simulink model "seat_heating_control"  (R2023b)
settings: Solver=FixedStepDiscrete  StartTime=0.0  StopTime=10.0  FixedStep=0.01  RelTol=1e-3
values from neighbouring files (symbols this model uses):
  RTE_OK = 0    [init.m]
  TemperatureStage1 = Simulink.Parameter    [init.m]
  TemperatureStage2 = Simulink.Parameter    [init.m]
  TemperatureStage3 = Simulink.Parameter    [init.m]
undefined symbols (not defined in the file or in its folder): EnumPowerState
settings Model: Creator=nabilekhoury  LastModifiedBy=developer
settings SolverCC: AlgebraicLoopSolver=TrustRegion
settings DataIOCC: SaveFormat=StructureWithTime
settings OptimizationCC: DefaultParameterBehavior=Inlined  EnhancedBackFolding=on  MemcpyThreshold=640  PassReuseOutputArgsAs=Individual arguments  ZeroExternalMemoryAtStartup=off  ZeroInternalMemoryAtStartup=off  InitFltsAndDblsToZero=on  OptimizeBlockOrder=speed  DifferentSizesBufferReuse=on  OptimizationCustomize=off  EfficientTunableParamExpr=on
settings DebuggingCC: ParameterTunabilityLossMsg=error  UnconnectedInputMsg=warning  UnconnectedOutputMsg=warning  UnconnectedLineMsg=warning  ArithmeticOperatorsInVariantConditions=warning
settings ModelReferenceCC: EnableRefExpFcnMdlSchedulingChecks=on  ModelReferenceNumInstancesAllowed=Single
settings SFSimCC: MATLABDynamicMemAlloc=off  CustomCodeUndefinedFunction=UseInterfaceOnly
settings RTWCC: Description=Embedded Coder  SystemTargetFile=ert.tlc  GenCodeOnly=on  TemplateMakefile=ert_default_tmf  IncludeHyperlinkInReport=on
settings CodeAppCC: ForceParamTrailComments=on  IgnoreCustomStorageClasses=off  OperatorAnnotations=on  SimulinkDataObjDesc=on  SFDataObjDesc=on  InsertBlockDesc=on
settings ERTTargetCC: TargetLangStandard=C99 (ISO)  GenerateSampleERTMain=on  SupportAbsoluteTime=off  SupportNonFinite=off  SupportComplex=off  InlinedParameterPlacement=NonHierarchical  ERTCustomFileTemplate=example_file_process.tlc

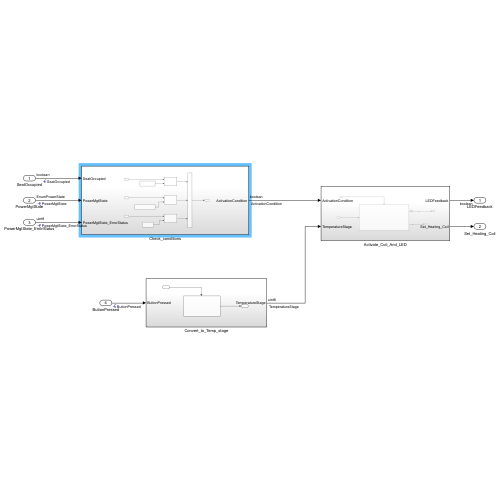
[thumbnail: Simulink's stored preview of the top-level diagram]
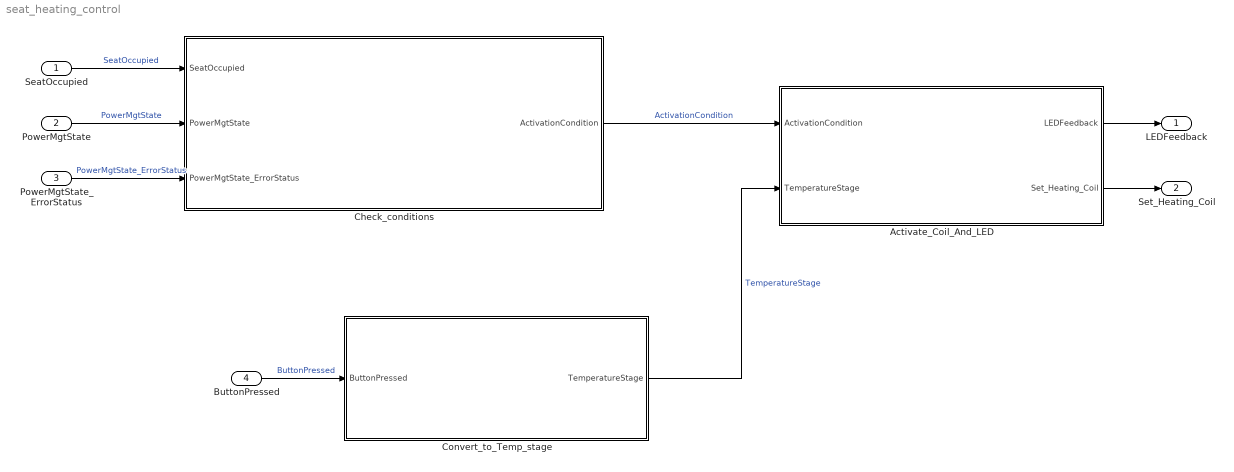
== system seat_heating_control ==
  SeatOccupied : Inport  OutDataTypeStr=boolean  PortDimensions=1
  PowerMgtState : Inport  Port=2  OutDataTypeStr=Enum: EnumPowerState  PortDimensions=1
  PowerMgtState_ErrorStatus : Inport  Port=3  OutDataTypeStr=uint8  PortDimensions=1
  ButtonPressed : Inport  Port=4
  Activate_Coil_And_LED : Subsystem
  Check_conditions : Subsystem
  Convert_to_Temp_stage : Subsystem
  LEDFeedback : Outport  OutDataTypeStr=boolean
  Set_Heating_Coil : Outport  Port=2
  wires:
  SeatOccupied/1 -> Check_conditions/1(SeatOccupied)  "SeatOccupied"
  PowerMgtState/1 -> Check_conditions/2(PowerMgtState)  "PowerMgtState"
  PowerMgtState_ErrorStatus/1 -> Check_conditions/3(PowerMgtState_ErrorStatus)  "PowerMgtState_ErrorStatus"
  Activate_Coil_And_LED/1(LEDFeedback) -> LEDFeedback/1
  Convert_to_Temp_stage/1(TemperatureStage) -> Activate_Coil_And_LED/2(TemperatureStage)  "TemperatureStage"
  Check_conditions/1(ActivationCondition) -> Activate_Coil_And_LED/1(ActivationCondition)  "ActivationCondition"
  ButtonPressed/1 -> Convert_to_Temp_stage/1(ButtonPressed)  "ButtonPressed"
  Activate_Coil_And_LED/2(Set_Heating_Coil) -> Set_Heating_Coil/1

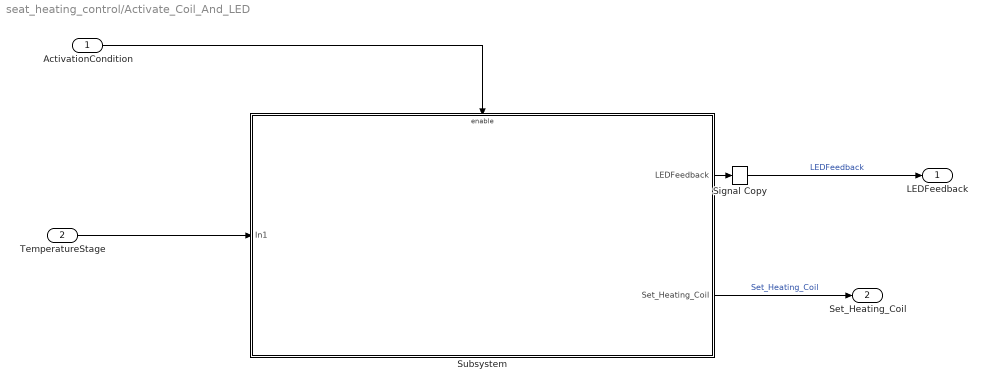
== system seat_heating_control/Activate_Coil_And_LED ==
  ActivationCondition : Inport
  TemperatureStage : Inport  Port=2
  Signal Copy : SignalConversion  OverrideOpt=off
  Subsystem : Subsystem
  LEDFeedback : Outport
      settings: EnsureOutportIsVirtual=on
  Set_Heating_Coil : Outport  Port=2
  wires:
  ActivationCondition/1 -> Subsystem/Enable
  TemperatureStage/1 -> Subsystem/1(In1)
  Subsystem/1(LEDFeedback) -> Signal Copy/1
  Subsystem/2(Set_Heating_Coil) -> Set_Heating_Coil/1  "Set_Heating_Coil"
  Signal Copy/1 -> LEDFeedback/1  "LEDFeedback"

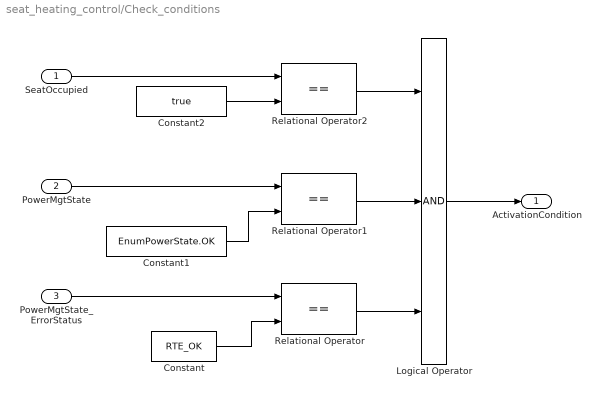
== system seat_heating_control/Check_conditions ==
  SeatOccupied : Inport
  PowerMgtState : Inport  Port=2
  PowerMgtState_ErrorStatus : Inport  Port=3
  Constant : Constant  Value=RTE_OK
  Constant1 : Constant  Value=EnumPowerState.OK
  Constant2 : Constant  Value=true
  Logical Operator : Logic  Inputs=3  AllPortsSameDT=off  OutDataTypeStr=boolean
  Relational Operator : RelationalOperator  Operator===  OutDataTypeStr=boolean  RndMeth=Simplest  InputSameDT=off
  Relational Operator1 : RelationalOperator  Operator===  OutDataTypeStr=boolean  RndMeth=Simplest  InputSameDT=off
  Relational Operator2 : RelationalOperator  Operator===  OutDataTypeStr=boolean  RndMeth=Simplest  InputSameDT=off
  ActivationCondition : Outport  OutDataTypeStr=boolean  PortDimensions=1  InitialOutput=0
  wires:
  Logical Operator/1 -> ActivationCondition/1
  PowerMgtState_ErrorStatus/1 -> Relational Operator/1
  PowerMgtState/1 -> Relational Operator1/1
  Constant2/1 -> Relational Operator2/2
  SeatOccupied/1 -> Relational Operator2/1
  Relational Operator2/1 -> Logical Operator/1
  Constant1/1 -> Relational Operator1/2
  Relational Operator/1 -> Logical Operator/3
  Relational Operator1/1 -> Logical Operator/2
  Constant/1 -> Relational Operator/2

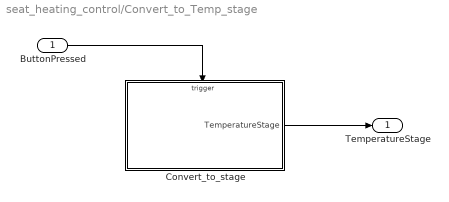
== system seat_heating_control/Convert_to_Temp_stage ==
  ButtonPressed : Inport
  Convert_to_stage : Subsystem
  TemperatureStage : Outport  OutDataTypeStr=uint8  PortDimensions=1  InitialOutput=0
  wires:
  Convert_to_stage/1(TemperatureStage) -> TemperatureStage/1
  ButtonPressed/1 -> Convert_to_stage/Trigger

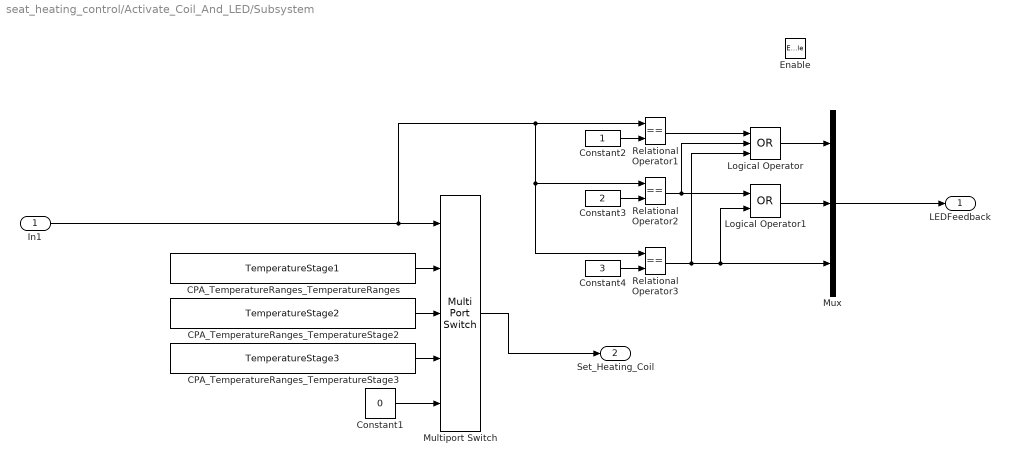
== system seat_heating_control/Activate_Coil_And_LED/Subsystem ==
  In1 : Inport
  Enable : EnablePort
  CPA_TemperatureRanges_TemperatureRanges : Constant  Value=TemperatureStage1
  CPA_TemperatureRanges_TemperatureStage2 : Constant  Value=TemperatureStage2
  CPA_TemperatureRanges_TemperatureStage3 : Constant  Value=TemperatureStage3
  Constant1 : Constant  Value=0
  Constant2 : Constant  OutDataTypeStr=Inherit: Inherit via back propagation
  Constant3 : Constant  Value=2  OutDataTypeStr=Inherit: Inherit via back propagation
  Constant4 : Constant  Value=3  OutDataTypeStr=Inherit: Inherit via back propagation
  Logical Operator : Logic  Operator=OR  Inputs=3  AllPortsSameDT=off  OutDataTypeStr=boolean
  Logical Operator1 : Logic  Operator=OR  AllPortsSameDT=off  OutDataTypeStr=boolean
  Multiport Switch : MultiPortSwitch  DataPortIndices={0,1,2,3}  DataPortForDefault=Additional data port  DiagnosticForDefault=None  OutDataTypeStr=uint8  SaturateOnIntegerOverflow=off  InputSameDT=off
  Mux : Mux  Inputs=3
  Relational Operator1 : RelationalOperator  Operator===  OutDataTypeStr=boolean  RndMeth=Simplest  InputSameDT=off
  Relational Operator2 : RelationalOperator  Operator===  OutDataTypeStr=boolean  RndMeth=Simplest  InputSameDT=off
  Relational Operator3 : RelationalOperator  Operator===  OutDataTypeStr=boolean  RndMeth=Simplest  InputSameDT=off
  LEDFeedback : Outport
  Set_Heating_Coil : Outport  Port=2
  wires:
  In1/1 -> Relational Operator3/1, Relational Operator2/1, Relational Operator1/1, Multiport Switch/1
  Constant2/1 -> Relational Operator1/2
  Constant4/1 -> Relational Operator3/2
  Mux/1 -> LEDFeedback/1
  CPA_TemperatureRanges_TemperatureStage2/1 -> Multiport Switch/3
  Relational Operator2/1 -> Logical Operator1/1, Logical Operator/2
  Relational Operator1/1 -> Logical Operator/1
  Constant3/1 -> Relational Operator2/2
  Relational Operator3/1 -> Logical Operator/3, Logical Operator1/2, Mux/3
  Multiport Switch/1 -> Set_Heating_Coil/1
  Constant1/1 -> Multiport Switch/5
  CPA_TemperatureRanges_TemperatureStage3/1 -> Multiport Switch/4
  CPA_TemperatureRanges_TemperatureRanges/1 -> Multiport Switch/2
  Logical Operator/1 -> Mux/1
  Logical Operator1/1 -> Mux/2

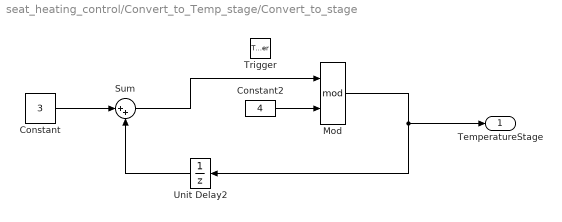
== system seat_heating_control/Convert_to_Temp_stage/Convert_to_stage ==
  Trigger : TriggerPort  VariantControl=Variant  PortDimensions=1
  Constant : Constant  Value=3  OutDataTypeStr=Inherit: Inherit via back propagation
  Constant2 : Constant  Value=4  OutDataTypeStr=Inherit: Inherit via back propagation
  Mod : Math  Operator=mod
  Sum : Sum  Inputs=|++
  Unit Delay2 : UnitDelay  SampleTime=-1  HasFrameUpgradeWarning=on
      settings: AttributesFormatString=Init = %<InitialCondition>
  TemperatureStage : Outport  InitialOutput=0
  wires:
  Sum/1 -> Mod/1
  Constant/1 -> Sum/1
  Mod/1 -> TemperatureStage/1, Unit Delay2/1
  Constant2/1 -> Mod/2
  Unit Delay2/1 -> Sum/2
